simulink model "ADC"  (Simulink 10.2)
settings: Solver=FixedStepAuto  StartTime=0.0  StopTime=0.04  FixedStep=1e-6  RelTol=1e-3
settings Model: Creator=YiboWang  LastModifiedBy=YiboWang
settings DataIOCC: SaveFormat=Dataset  SignalLoggingSaveFormat=Dataset  ReturnWorkspaceOutputs=on
settings OptimizationCC: LifeSpan=auto
settings DebuggingCC: UnderspecifiedInitializationDetection=Simplified  MergeDetectMultiDrivingBlocksExec=error  FcnCallInpInsideContextMsg=error  SFUnexpectedBacktrackingDiag=error  SFNoUnconditionalDefaultTransitionDiag=error  SFExecutionAtInitializationDiag=warning  ArithmeticOperatorsInVariantConditions=error
settings HardwareCC: ProdBitPerPointer=64  ProdBitPerSizeT=64  ProdBitPerPtrDiffT=64  ProdLargestAtomicFloat=Float  ProdIntDivRoundTo=Zero  ProdEndianess=LittleEndian  ProdWordSize=64  ProdHWDeviceType=Intel->x86-64 (Windows64)
settings ModelReferenceCC: PropagateSignalLabelsOutOfModel=on
settings SFSimCC: SimUseLocalCustomCode=on  CustomCodeUndefinedFunction=FilterOut
settings RTWCC: RTWUseLocalCustomCode=on
settings CodeAppCC: StateflowObjectComments=off
settings GRTTargetCC: TargetLangStandard=C99 (ISO)  CombineOutputUpdateFcns=on  GRTInterface=off
settings ConfigComp: CovMetricSettings=dwe  CovSaveCumulativeToWorkspaceVar=off  CovSaveSingleToWorkspaceVar=off  CovExternalEMLEnable=on

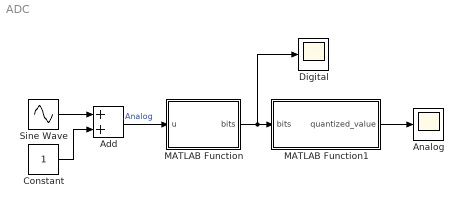
== system ADC ==
  Add : Sum
  Analog : Scope
  Constant : Constant
  Digital : Scope
  MATLAB Function : MATLAB Function  TreatAsAtomicUnit=on
  MATLAB Function1 : MATLAB Function  TreatAsAtomicUnit=on
  Sine Wave : Sin  Frequency=2*pi*50  SampleTime=0
  wires:
  MATLAB Function/1(bits) -> Digital/1, MATLAB Function1/1(bits)
  Sine Wave/1 -> Add/1
  Add/1 -> MATLAB Function/1(u)  "Analog"
  Constant/1 -> Add/2
  MATLAB Function1/1(quantized_value) -> Analog/1

== matlab function MATLAB Function1 ==
  data: bits input double; quantized_value output double
function quantized_value = adc_reconstruction(bits)
% 权重数组（MSB到LSB）
weights = 2.^(7:-1:0)';  % [128;64;32;16;8;4;2;1]

% 计算量化值
quantized_value = double(bits) * weights / 255;
end

== matlab function MATLAB Function ==
  data: u input double; bits output double
function bits = adc_function(u)
% 8-bit ADC转换函数
% 输入：
%   u - 模拟输入信号（假设范围0-1）
% 输出：
%   bits - 8位二进制数组（MSB到LSB排列）

% 定义参考电压（根据实际信号范围调整）
Vref = 2;

% 信号缩放和数字化
scaled_value = (u / Vref) * 255;          % 缩放信号到0-255范围
digital_code = round(scaled_value);       % 四舍五入量化
digital_code = uint8(max(0, min(255, digital_code))); % 钳位并转换为uint8

% 二进制位提取（MSB到LSB）
bits = zeros(1,8,'uint8');
for i = 1:8
    bits(i) = bitget(digital_code, 9-i);  % 提取从高位到低位
end
end
